simulink model "ecualizador"  (Simulink 9.3)
settings: Solver=ode45  StartTime=0.0  StopTime=50  RelTol=1e-3  EnableMultiTasking=on
libraries: dsparch4 x3, simulink x3, dspvision x1, dspobslib x1
settings Model: Creator=Rafael Bustamante  LastModifiedBy=JORGE
settings DataIOCC: LimitDataPoints=on  SignalLoggingSaveFormat=Dataset
settings DebuggingCC: UnderspecifiedInitializationDetection=Simplified  MergeDetectMultiDrivingBlocksExec=error  FcnCallInpInsideContextMsg=error
settings GRTTargetCC: GeneratePreprocessorConditionals=Disable all  CombineOutputUpdateFcns=on  GRTInterface=off

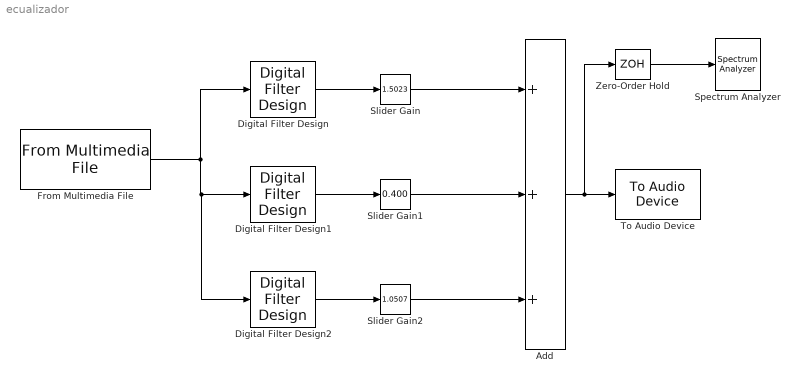
== system ecualizador ==
  Add : Sum  Inputs=+++  AccumDataTypeStr=double
  Digital Filter Design : dsparch4/Digital Filter Design  mwdsp_browser_bugfix_var=off
  Digital Filter Design1 : dsparch4/Digital Filter Design  mwdsp_browser_bugfix_var=off
  Digital Filter Design2 : dsparch4/Digital Filter Design  mwdsp_browser_bugfix_var=off
  From Multimedia File : dspvision/From Multimedia File  inputFilename=C:\Users\JORGE\Downloads\06 Love Maze.wav  readRange=[1 Inf]  loop=on  numPlays=inf  outputStreams=Audio only  videoDataType=single  audioDataType=double  inheritSampleTime=on  userDefinedSampleTime=1/30  noAudioOutput=off  isIntensityVideo=off  fourcc=RGB  colorVideoFormat=Separate color signals  outputEOF=off  dataOrg=Column-major  audioFrameSize=1024  computeAudioFrameSize=off  outSamplingMode=Frame based
      settings: SourceProductName=DSP System Toolbox  SourceProductBaseCode=DS
  Slider Gain : simulink/Math Operations/Slider Gain  gain=1.5023  low=0  high=2
  Slider Gain1 : simulink/Math Operations/Slider Gain  gain=0.400  low=0  high=2
  Slider Gain2 : simulink/Math Operations/Slider Gain  gain=1.0507  low=0  high=2
  Spectrum Analyzer : SpectrumAnalyzer
  To Audio Device : dspobslib/To Audio Device  deviceName=Default  inheritSampleRate=on  sampleRate=44100  deviceDatatype=Determine from input data type  autoBufferSize=on  bufferSize=4096  queueDuration=1.0  defaultOutputChannelMapping=on  outputChannelMapping=1:2  outputNumUnderrunSamples=off
      settings: SourceProductName=DSP System Toolbox  SourceProductBaseCode=DS
  Zero-Order Hold : ZeroOrderHold  SampleTime=0.001
  wires:
  From Multimedia File/1 -> Digital Filter Design/1, Digital Filter Design2/1, Digital Filter Design1/1
  Digital Filter Design/1 -> Slider Gain/1
  Digital Filter Design1/1 -> Slider Gain1/1
  Digital Filter Design2/1 -> Slider Gain2/1
  Slider Gain/1 -> Add/1
  Slider Gain1/1 -> Add/2
  Slider Gain2/1 -> Add/3
  Add/1 -> Zero-Order Hold/1, To Audio Device/1
  Zero-Order Hold/1 -> Spectrum Analyzer/1
